simulink model "DCRemoval"  (R2014a)
settings: Solver=FixedStepDiscrete  StartTime=0.0  StopTime=3e+1  FixedStep=0.01  RelTol=1e-3
settings Model: Creator=hossein  LastModifiedBy=hossein

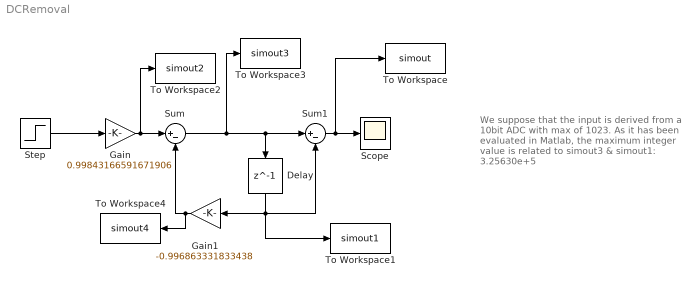
== system DCRemoval ==
  note: We suppose that the input is
      | derived from a 10bit ADC with
      | max of 1023.
      | As it has been evaluated in
      | Matlab, the maximum integer
      | value is related to simout3
      | & simout1: 3.25630e+5
  Delay : Delay  DelayLength=1  InitialCondition=0
  Gain : Gain  Gain=0.99843166591671906
  Gain1 : Gain  Gain=-0.996863331833438
  Scope : Scope
  Step : Step  After=511  SampleTime=0
  Sum : Sum  Inputs=|+-
  Sum1 : Sum  Inputs=|+-
  To Workspace : ToWorkspace  VariableName=simout  SampleTime=-1
      settings: Save2DSignal=2-D array (concatenate along first dimension)
  To Workspace1 : ToWorkspace  VariableName=simout1  SampleTime=-1
      settings: Save2DSignal=2-D array (concatenate along first dimension)
  To Workspace2 : ToWorkspace  VariableName=simout2  SampleTime=-1
      settings: Save2DSignal=2-D array (concatenate along first dimension)
  To Workspace3 : ToWorkspace  VariableName=simout3  SampleTime=-1
      settings: Save2DSignal=2-D array (concatenate along first dimension)
  To Workspace4 : ToWorkspace  VariableName=simout4  SampleTime=-1
      settings: Save2DSignal=2-D array (concatenate along first dimension)
  wires:
  Delay/1 -> To Workspace1/1, Sum1/2, Gain1/1
  Gain1/1 -> To Workspace4/1, Sum/2
  Gain/1 -> To Workspace2/1, Sum/1
  Step/1 -> Gain/1
  Sum/1 -> To Workspace3/1, Sum1/1, Delay/1
  Sum1/1 -> To Workspace/1, Scope/1
